simulink model "frequency_virt"  (Simulink 7.5)
settings: Solver=ode45  StartTime=0.0  StopTime=5  RelTol=1e-3
StopFcn:
  | save_system(vars.simfilename);
CloseFcn:
  | save_system(vars.simfilename); sim(vars.simfilename);vars.simtime = str2num(get_param(vars.simfilename,'StopTime'));set(guiel.hSimtime,'String',num2str(vars.simtime));if strcmp(vars.simfilename(end-2:end),'sim') vars.L= motorParams(1,1); vars.R= motorParams(1,2); vars.J= motorParams(1,3);vars.b= motorParams(1,4); vars.Kb= motorParams(1,5); vars.Km= motorParams(1,6);if (min(size(motorParams)) == 9) vars.P= motorParams(1,7); vars.I= motorParams(1,8); vars.D= motorParams(1,9);else;vars.P= NaN; vars.I= NaN; vars.D= NaN;end;clear motorParams; [vars.numericTF vars.symbolTF] = calcTF2(vars);end,
settings Model: Creator=Farid Golnaraghi  LastModifiedBy=Dan
settings DataIOCC: MaxDataPoints=10000
settings OptimizationCC: BlockReduction=off  BooleanDataType=off  InitFltsAndDblsToZero=on
settings DebuggingCC: SaveWithParameterizedLinksMsg=none  SignalResolutionControl=TryResolveAllWithWarning  SolverPrmCheckMsg=none  MultiTaskDSMMsg=warning  MultiTaskCondExecSysMsg=none  StrictBusMsg=None
settings HardwareCC: TargetUnknown=on
settings RTWCC: IncludeERTFirstTime=on
settings GRTTargetCC: TargetFcnLib=ansi_tfl_tmw.mat

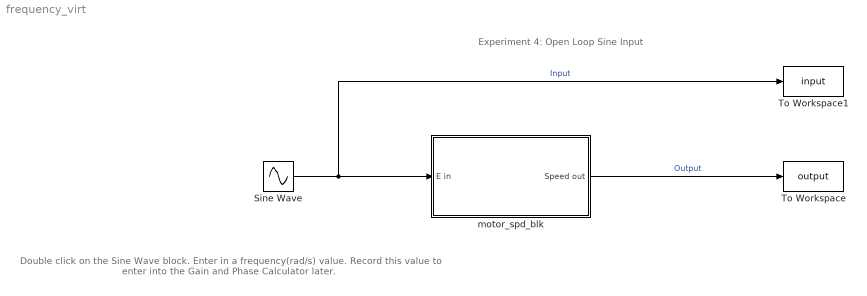
== system frequency_virt ==
  note: Experiment 4: Open Loop Sine Input
  note: Double click on the Sine Wave block.
      | Enter in a frequency(rad/s) value.
      | Record this value to enter into the
      | Gain and Phase Calculator later.
  Sine Wave : Sin  Amplitude=1  Bias=0  Frequency=0.1*2*pi  Phase=0  Samples=10  SampleTime=0  Offset=0
  To Workspace : ToWorkspace  VariableName=output  SampleTime=-1  SaveFormat=Structure With Time
  To Workspace1 : ToWorkspace  VariableName=input  SampleTime=-1  SaveFormat=Structure With Time
  motor_spd_blk : Subsystem
      mask Description: Real-Time Workshop generated S-function.
      mask Help: web(['file://',docroot,'/toolbox/rtw/rtwsfcn.html']);
      mask Display: disp('DC Motor (Speed Control)')
  wires:
  motor_spd_blk/1(Speed out) -> To Workspace/1  "Output"
  Sine Wave/1 -> To Workspace1/1, motor_spd_blk/1(E in)  "Input"

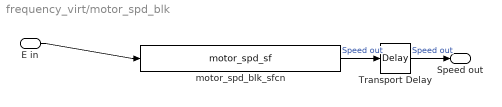
== system frequency_virt/motor_spd_blk ==
  E in : Inport  OutDataType=sfix(16)  OutScaling=2^0
  Transport Delay : TransportDelay  DelayTime=0.001
  motor_spd_blk_sfcn : S-Function  FunctionName=motor_spd_sf  SFunctionModules=""  EnableBusSupport=off  mask{rtw_sf_name=motor_spd_sf, showVar=off}
      mask prompts: rtw_sf_name "Generated S-function name (model_sf):"; showVar "Show module list"
      mask help: Real-Time Workshop generated S-function.
      mask init:
      | displist = '';
      | if ~strcmp(get_param(gcb, 'FunctionName'), rtw_sf_name);
      |   set_param(gcb, 'FunctionName', rtw_sf_name);
      | end
      | if  showVar & exist('rtwsfunc') == 2
      |   tmplist = rtwsfunc(rtw_sf_name,gcb);
      |   tmplist = ['\nList of Modules:\n', tmplist];
      | elseif showVar
      |   tmplist = '\nList of Modules:\nRTW not licensed\n';
      | end
      | if showVar
      |   displist = tmplist;
      | end
      settings: CopyFcn=set_param(gcb,'linkstatus','none')
      mask Help: web(['file://',docroot,'/toolbox/rtw/rtwsfcn.html']);
      mask Display:
      | port_label('input',1,'E in');
      | port_label('output',1,'Speed out');
  Speed out : Outport  OutDataType=sfix(16)  OutScaling=2^0
  wires:
  Transport Delay/1 -> Speed out/1  "Speed out"
  motor_spd_blk_sfcn/1 -> Transport Delay/1  "Speed out"
  E in/1 -> motor_spd_blk_sfcn/1
